simulink model "Blank_Controller_1"  (Simulink 7.5)
settings: Solver=ode45  StartTime=0.0  StopTime=10.0  RelTol=1e-3
settings Model: Creator=sriddle  LastModifiedBy=sriddle

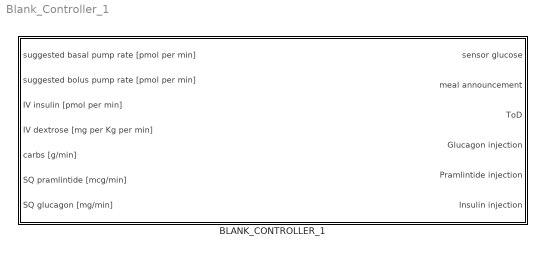
== system Blank_Controller_1 ==
  BLANK_CONTROLLER_1 : Subsystem

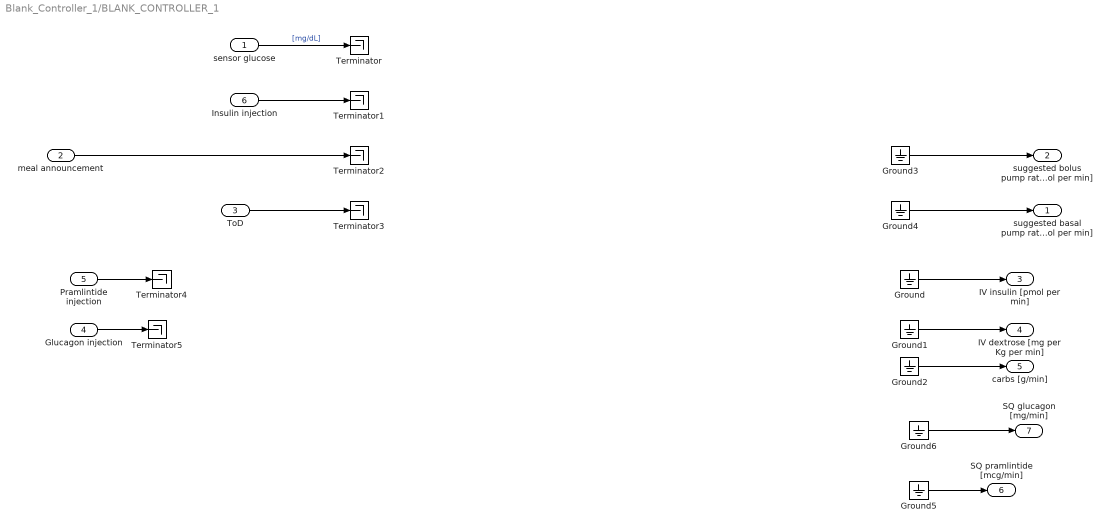
== system Blank_Controller_1/BLANK_CONTROLLER_1 ==
  sensor glucose : Inport  OutDataType=sfix(16)  OutScaling=2^0
  meal announcement : Inport  Port=2  OutDataType=sfix(16)  OutScaling=2^0
  ToD : Inport  Port=3  OutDataType=sfix(16)  OutScaling=2^0
  Glucagon injection : Inport  Port=4
  Pramlintide injection : Inport  Port=5
  Insulin injection : Inport  Port=6  OutDataType=sfix(16)  OutScaling=2^0
  Ground{,1..6} (7 alike) : Ground
  Terminator{,1..5} (6 alike) : Terminator
  suggested basal pump rate [pmol per min] : Outport  OutDataType=sfix(16)  OutScaling=2^0
  suggested bolus pump rate [pmol per min] : Outport  Port=2  OutDataType=sfix(16)  OutScaling=2^0
  IV insulin [pmol per min] : Outport  Port=3  OutDataType=sfix(16)  OutScaling=2^0
  IV dextrose [mg per Kg per min] : Outport  Port=4  OutDataType=sfix(16)  OutScaling=2^0
  carbs [g/min] : Outport  Port=5  OutDataType=sfix(16)  OutScaling=2^0
  SQ pramlintide [mcg/min] : Outport  Port=6
  SQ glucagon [mg/min] : Outport  Port=7
  wires:
  Ground2/1 -> carbs [g/min]/1
  Ground1/1 -> IV dextrose [mg per Kg per min]/1
  Ground/1 -> IV insulin [pmol per min]/1
  Ground4/1 -> suggested basal pump rate [pmol per min]/1
  Ground3/1 -> suggested bolus pump rate [pmol per min]/1
  sensor glucose/1 -> Terminator/1  "[mg/dL]"
  Insulin injection/1 -> Terminator1/1
  ToD/1 -> Terminator3/1
  meal announcement/1 -> Terminator2/1
  Pramlintide injection/1 -> Terminator4/1
  Glucagon injection/1 -> Terminator5/1
  Ground6/1 -> SQ glucagon [mg/min]/1
  Ground5/1 -> SQ pramlintide [mcg/min]/1
